simulink model "RL_multi_control_system"  (R2021a)
settings: Solver=ode23t  StartTime=0.0  StopTime=10.0  RelTol=1e-3  AbsTol=1e-3
undefined symbols (not defined in the file or in its folder): dphi0, dtheta0, phi0, Tf, theta0, Ts
libraries: angle_lib x8, rllib x2, simulink x2, pendulumLib x1
settings Model: DataDictionary=rl_data.sldd  Creator=tshintai  LastModifiedBy=THMOS
settings SolverCC: AutoScaleAbsTol=off
settings ExplorerConfigSet: InternalSimMechanicsExplorerSettings="<ExplorerConfiguration><canonicalview>default</canonicalview><AnimationSetting><BasePlaybackSpeed>1.0</BasePlaybackSpeed><PlaybackSpeedFactor>1.0</PlaybackSpeedFactor></AnimationSetting><TilePanel><TileInfo><Tiles Columns=\"1\" Count=\"1\" Rows=\"1\"><Column Weight=\"1\"/><Row Weight=\"1\"/><Tile Height=\"1\" Width=\"1\" X=\"0\" Y=\"0\"/></Tiles></TileInfo><SceneInfo><SceneViewer><BGColor><R>0.60000002384185791</R><G>0.60000002384185791</G><B>0.60000002384185791</B></BGColor><Camera><DoPerspective>on</DoPerspective><Position><X>0.334156231583514596</X><Y>0.107146061295956732</Y><Z>0.154419804164132285</Z></Position><Center><X>0.145480827141795971</X><Y>0.0537418892551446009</Y><Z>0.077934111254939889</Z></Center><Up><X>-0.332530024195597795</X><Y>-0.157027945704575345</Y><Z>0.929927958110882913</Z></Up><ViewLimDist>1</ViewLimDist><YLim>0.466307658154998583</YLim><XLim>0.535390274177961367</XLim></Camera></SceneViewer></SceneInfo></TilePanel><MechEditorPanel><Cameras><Camera><Id>Camera1</Id><Value><Name>Camera1</Name><NativeCamera><PositionKeyframeSet/><CenterKeyframeSet/><UpVectorKeyframeSet/></NativeCamera></Value></Camera></Cameras><GfxPanelCameraMap><MapElement CameraMLId=\"Camera1\" GfxPanelIndex=\"0\"/></GfxPanelCameraMap><VideoCreator><PlaybackSpeedRatio>1.0</PlaybackSpeedRatio><FrameRate>30</FrameRate><VideoFormat>Motion JPEG AVI</VideoFormat><FrameSize>auto</FrameSize></VideoCreator></MechEditorPanel></ExplorerConfiguration>"

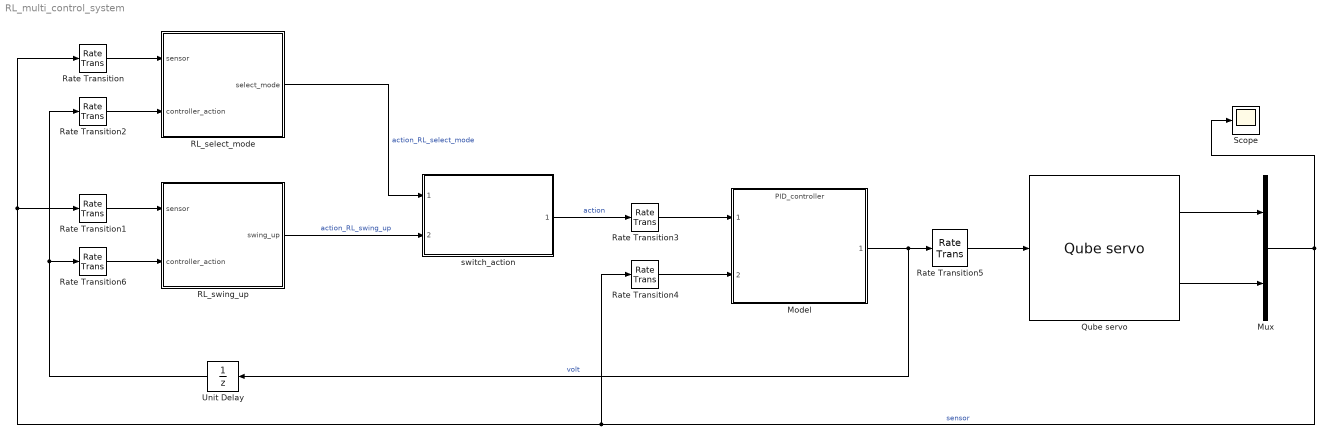
== system RL_multi_control_system ==
  Model : ModelReference  ModelNameDialog=PID_controller.slx  SimulationMode=Normal  ModelReferenceVersion=2.2
  Mux : Mux  Inputs=2
  Qube servo : pendulumLib/Qube servo  a0=[theta0, phi0]  w0=[dtheta0, dphi0]  R_m=R_m  L_m=L_m  mu_m=mu_m  K_b=K_b_2  n=n  rod_mass=m_r  rod_length=L_r  rod_rad=rod_rad  p_mass=m_p  p_length=L_p  p_rad=p_rad  D_r=D_r_2  D_p=D_p
  RL_select_mode : Subsystem
  RL_swing_up : Subsystem
  Rate Transition{,1..2,6} (4 alike) : RateTransition  OutPortSampleTime=Ts
  Rate Transition3 : RateTransition  OutPortSampleTime=Tc
  Rate Transition4 : RateTransition  OutPortSampleTime=Tc
  Rate Transition5 : RateTransition
  Scope : Scope
  Unit Delay : UnitDelay  SampleTime=-1  HasFrameUpgradeWarning=on
  switch_action : Subsystem  ReferencedSubsystem=RL_multi_switch_action
  wires:
  Qube servo/1 -> Mux/1
  Qube servo/2 -> Mux/2
  Mux/1 -> Rate Transition1/1, Rate Transition/1, Rate Transition4/1, Scope/1  "sensor"
  Rate Transition4/1 -> Model/2
  Model/1 -> Rate Transition5/1, Unit Delay/1  "volt"
  Rate Transition5/1 -> Qube servo/1
  Rate Transition3/1 -> Model/1
  Unit Delay/1 -> Rate Transition6/1, Rate Transition2/1
  RL_swing_up/1(swing_up) -> switch_action/2  "action_RL_swing_up"
  switch_action/1 -> Rate Transition3/1  "action"
  RL_select_mode/1(select_mode) -> switch_action/1  "action_RL_select_mode"
  Rate Transition/1 -> RL_select_mode/1(sensor)
  Rate Transition2/1 -> RL_select_mode/2(controller_action)
  Rate Transition1/1 -> RL_swing_up/1(sensor)
  Rate Transition6/1 -> RL_swing_up/2(controller_action)

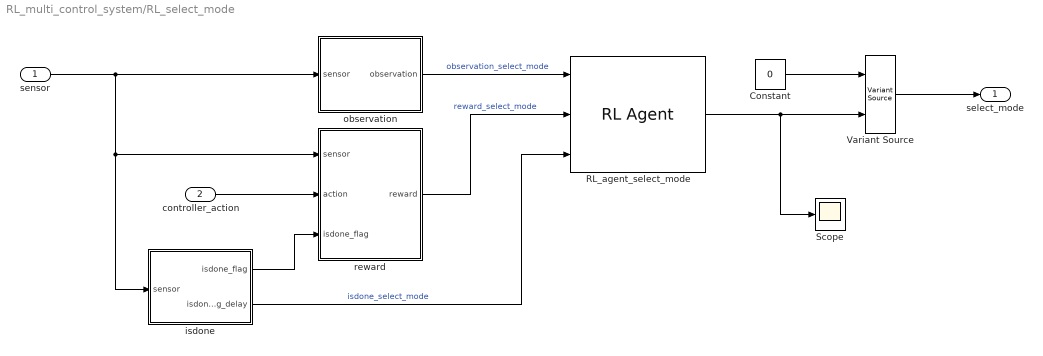
== system RL_multi_control_system/RL_select_mode ==
  sensor : Inport
  controller_action : Inport  Port=2
  Constant : Constant  Value=0
  RL_agent_select_mode : rllib/RL Agent  Agent=agent_select  ExternalActionAsInput=off  ProvideCumRwd=off  TreatAsDirectFeedthrough=on
  Scope : Scope
  Variant Source : VariantSource
  isdone : Subsystem  VariantControl=VARIANT_INV_POS
  "observation " : Subsystem  VariantControl=VARIANT_OBS_ARM_PEND
  reward : Subsystem  VariantControl=VARIANT_INV_POS
  select_mode : Outport
  wires:
  RL_agent_select_mode/1 -> Scope/1, Variant Source/2
  "observation "/1(observation) -> RL_agent_select_mode/1  "observation_select_mode"
  reward/1(reward) -> RL_agent_select_mode/2  "reward_select_mode"
  controller_action/1 -> reward/2(action)
  isdone/2(isdone_flag_delay) -> RL_agent_select_mode/3  "isdone_select_mode"
  sensor/1 -> "observation "/1(sensor), isdone/1(sensor), reward/1(sensor)
  isdone/1(isdone_flag) -> reward/3(isdone_flag)
  Variant Source/1 -> select_mode/1
  Constant/1 -> Variant Source/1

== system RL_multi_control_system/RL_swing_up ==
  sensor : Inport
  controller_action : Inport  Port=2
  Gain : Gain  Gain=3*pi/4
  RL_agent_swing_up : rllib/RL Agent  Agent=agent_swing  ExternalActionAsInput=off  ProvideCumRwd=off  TreatAsDirectFeedthrough=on
  isdone : Subsystem  VariantControl=VARIANT_INV_POS
  "observation " : Subsystem  VariantControl=VARIANT_OBS_ARM_PEND
  reward : Subsystem  VariantControl=VARIANT_INV_POS
  swing_up : Outport
  wires:
  isdone/1(isdone_flag) -> reward/3(isdone_flag)
  sensor/1 -> "observation "/1(sensor), isdone/1(sensor), reward/1(sensor)
  isdone/2(isdone_flag_delay) -> RL_agent_swing_up/3  "isdone_swing_up"
  controller_action/1 -> reward/2(action)
  reward/1(reward) -> RL_agent_swing_up/2  "reward_swing_up"
  "observation "/1(observation) -> RL_agent_swing_up/1  "observation_swing_up"
  RL_agent_swing_up/1 -> Gain/1
  Gain/1 -> swing_up/1

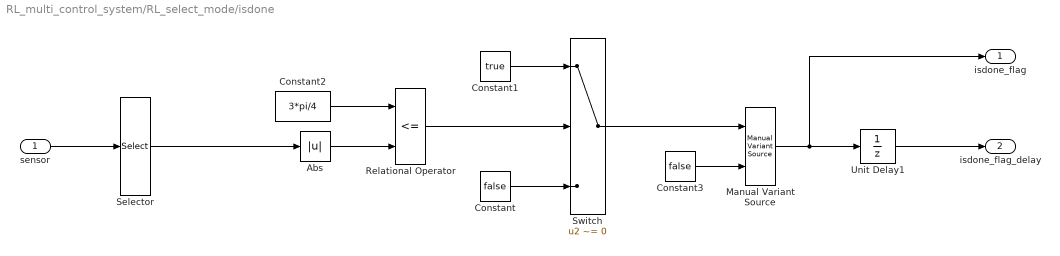
== system RL_multi_control_system/RL_select_mode/isdone ==
  sensor : Inport
  Abs : Abs
  Constant : Constant  Value=false
  Constant1 : Constant  Value=true
  Constant2 : Constant  Value=3*pi/4
  Constant3 : Constant  Value=false
  Manual Variant Source : simulink/Signal Routing/Manual Variant Source  NumChoices=2  LabelModeActiveChoice=V_2
  Relational Operator : RelationalOperator  Operator=<=  OutDataTypeStr=boolean  RndMeth=Simplest
  Selector : Selector  InputPortWidth=4  IndexOptions=Index vector (dialog)  Indices=[1]  OutputSizes=1
  Switch : Switch  Criteria=u2 ~= 0
  Unit Delay1 : UnitDelay  SampleTime=-1  HasFrameUpgradeWarning=on
  isdone_flag : Outport
  isdone_flag_delay : Outport  Port=2
  wires:
  Unit Delay1/1 -> isdone_flag_delay/1
  Constant3/1 -> Manual Variant Source/2
  Manual Variant Source/1 -> Unit Delay1/1, isdone_flag/1
  Switch/1 -> Manual Variant Source/1
  Selector/1 -> Abs/1
  Constant1/1 -> Switch/1
  Abs/1 -> Relational Operator/2
  Relational Operator/1 -> Switch/2
  Constant/1 -> Switch/3
  Constant2/1 -> Relational Operator/1
  sensor/1 -> Selector/1

== system RL_multi_control_system/RL_select_mode/observation  ==
  sensor : Inport
  Demux : Demux
  Mux : Mux  Inputs=6
  Trigonometric Function : Trigonometry
  Trigonometric Function1 : Trigonometry  Operator=cos
  Trigonometric Function2 : Trigonometry
  Trigonometric Function3 : Trigonometry  Operator=cos
  observation : Outport
  wires:
  Demux/3 -> Mux/5
  Demux/1 -> Trigonometric Function1/1, Trigonometric Function/1
  Trigonometric Function1/1 -> Mux/2
  Trigonometric Function/1 -> Mux/1
  Mux/1 -> observation/1  "observation"
  sensor/1 -> Demux/1
  Trigonometric Function2/1 -> Mux/3
  Trigonometric Function3/1 -> Mux/4
  Demux/2 -> Trigonometric Function3/1, Trigonometric Function2/1
  Demux/4 -> Mux/6

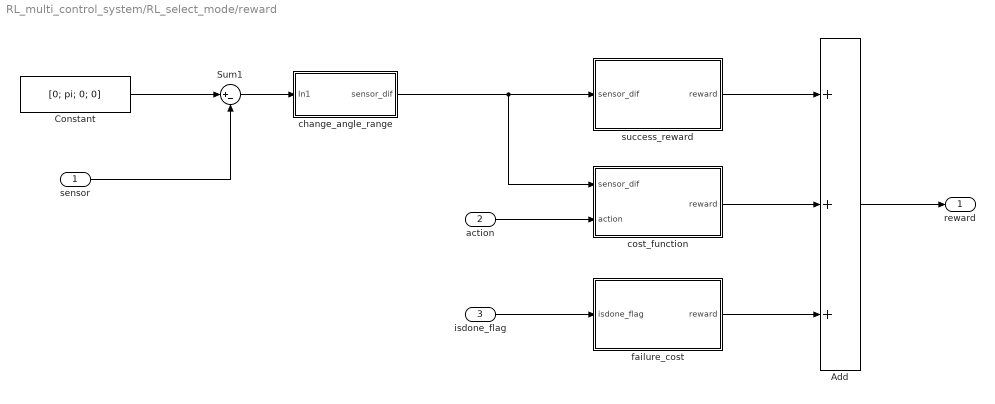
== system RL_multi_control_system/RL_select_mode/reward ==
  sensor : Inport
  action : Inport  Port=2
  isdone_flag : Inport  Port=3
  Add : Sum  Inputs=+++
  Constant : Constant  Value=[0; pi; 0; 0]
  Sum1 : Sum  Inputs=|+-
  change_angle_range : Subsystem
  cost_function : Subsystem
  failure_cost : Subsystem
  success_reward : Subsystem
  reward : Outport
  wires:
  isdone_flag/1 -> failure_cost/1(isdone_flag)
  failure_cost/1(reward) -> Add/3
  success_reward/1(reward) -> Add/1
  cost_function/1(reward) -> Add/2
  action/1 -> cost_function/2(action)
  Add/1 -> reward/1
  Sum1/1 -> change_angle_range/1(In1)
  sensor/1 -> Sum1/2
  Constant/1 -> Sum1/1
  change_angle_range/1(sensor_dif) -> success_reward/1(sensor_dif), cost_function/1(sensor_dif)

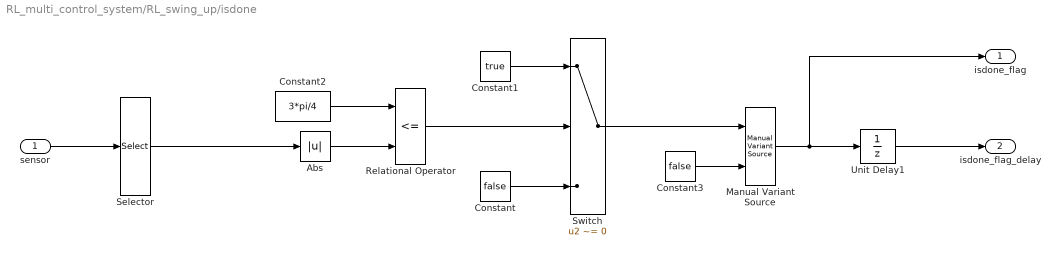
== system RL_multi_control_system/RL_swing_up/isdone ==
  sensor : Inport
  Abs : Abs
  Constant : Constant  Value=false
  Constant1 : Constant  Value=true
  Constant2 : Constant  Value=3*pi/4
  Constant3 : Constant  Value=false
  Manual Variant Source : simulink/Signal Routing/Manual Variant Source  NumChoices=2  LabelModeActiveChoice=V_2
  Relational Operator : RelationalOperator  Operator=<=  OutDataTypeStr=boolean  RndMeth=Simplest
  Selector : Selector  InputPortWidth=4  IndexOptions=Index vector (dialog)  Indices=[1]  OutputSizes=1
  Switch : Switch  Criteria=u2 ~= 0
  Unit Delay1 : UnitDelay  SampleTime=-1  HasFrameUpgradeWarning=on
  isdone_flag : Outport
  isdone_flag_delay : Outport  Port=2
  wires:
  sensor/1 -> Selector/1
  Constant2/1 -> Relational Operator/1
  Constant/1 -> Switch/3
  Relational Operator/1 -> Switch/2
  Abs/1 -> Relational Operator/2
  Constant1/1 -> Switch/1
  Selector/1 -> Abs/1
  Switch/1 -> Manual Variant Source/1
  Manual Variant Source/1 -> isdone_flag/1, Unit Delay1/1
  Constant3/1 -> Manual Variant Source/2
  Unit Delay1/1 -> isdone_flag_delay/1

== system RL_multi_control_system/RL_swing_up/observation  ==
  sensor : Inport
  Demux : Demux
  Mux : Mux  Inputs=6
  Trigonometric Function : Trigonometry
  Trigonometric Function1 : Trigonometry  Operator=cos
  Trigonometric Function2 : Trigonometry
  Trigonometric Function3 : Trigonometry  Operator=cos
  observation : Outport
  wires:
  Demux/4 -> Mux/6
  Demux/2 -> Trigonometric Function2/1, Trigonometric Function3/1
  Trigonometric Function3/1 -> Mux/4
  Trigonometric Function2/1 -> Mux/3
  sensor/1 -> Demux/1
  Mux/1 -> observation/1  "observation"
  Trigonometric Function/1 -> Mux/1
  Trigonometric Function1/1 -> Mux/2
  Demux/1 -> Trigonometric Function/1, Trigonometric Function1/1
  Demux/3 -> Mux/5

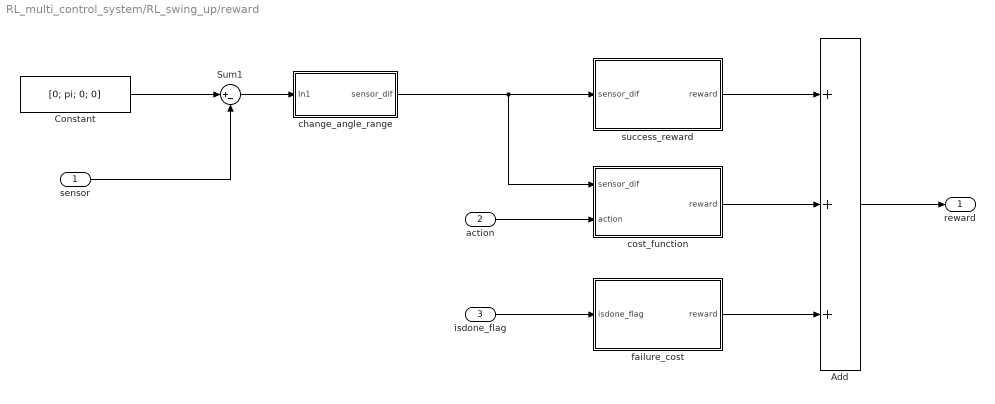
== system RL_multi_control_system/RL_swing_up/reward ==
  sensor : Inport
  action : Inport  Port=2
  isdone_flag : Inport  Port=3
  Add : Sum  Inputs=+++
  Constant : Constant  Value=[0; pi; 0; 0]
  Sum1 : Sum  Inputs=|+-
  change_angle_range : Subsystem
  cost_function : Subsystem
  failure_cost : Subsystem
  success_reward : Subsystem
  reward : Outport
  wires:
  isdone_flag/1 -> failure_cost/1(isdone_flag)
  failure_cost/1(reward) -> Add/3
  success_reward/1(reward) -> Add/1
  cost_function/1(reward) -> Add/2
  action/1 -> cost_function/2(action)
  Add/1 -> reward/1
  Sum1/1 -> change_angle_range/1(In1)
  sensor/1 -> Sum1/2
  Constant/1 -> Sum1/1
  change_angle_range/1(sensor_dif) -> success_reward/1(sensor_dif), cost_function/1(sensor_dif)

== system RL_multi_control_system/RL_select_mode/reward/change_angle_range ==
  In1 : Inport
  Demux : Demux
  Mux : Mux
  change_angle_range : angle_lib/change_angle_range  SystemSampleTime=-1  VariantActivationTime=update diagram  Latency=0  AutoFrameSizeCalculation=off
  change_angle_range1 : angle_lib/change_angle_range  SystemSampleTime=-1  VariantActivationTime=update diagram  Latency=0  AutoFrameSizeCalculation=off
  mod_2pi : angle_lib/mod_2pi  SystemSampleTime=-1  VariantActivationTime=update diagram  Latency=0  AutoFrameSizeCalculation=off
  mod_2pi1 : angle_lib/mod_2pi  SystemSampleTime=-1  VariantActivationTime=update diagram  Latency=0  AutoFrameSizeCalculation=off
  sensor_dif : Outport
  wires:
  mod_2pi1/1 -> change_angle_range1/1
  mod_2pi/1 -> change_angle_range/1
  Mux/1 -> sensor_dif/1
  Demux/4 -> Mux/4
  Demux/3 -> Mux/3
  change_angle_range1/1 -> Mux/2
  change_angle_range/1 -> Mux/1
  In1/1 -> Demux/1
  Demux/1 -> mod_2pi/1
  Demux/2 -> mod_2pi1/1

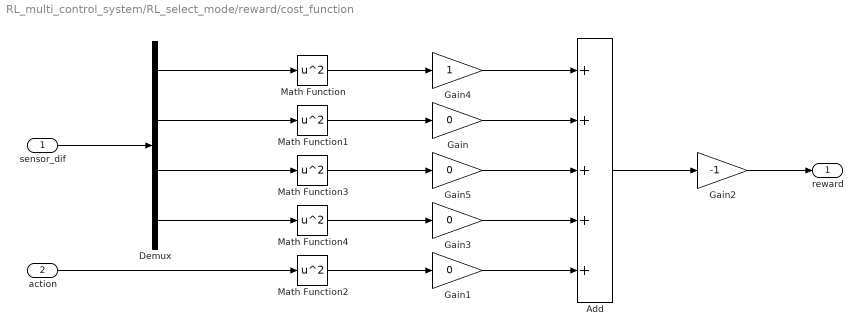
== system RL_multi_control_system/RL_select_mode/reward/cost_function ==
  sensor_dif : Inport
  action : Inport  Port=2
  Add : Sum  Inputs=+++++
  Demux : Demux
  Gain{,1,3,5} (4 alike) : Gain  Gain=0
  Gain2 : Gain  Gain=-1
  Gain4 : Gain
  Math Function{,1..4} (5 alike) : Math  Operator=square  SaturateOnIntegerOverflow=on
  reward : Outport
  wires:
  Math Function4/1 -> Gain3/1
  Gain4/1 -> Add/1
  Gain/1 -> Add/2
  Gain5/1 -> Add/3
  Gain3/1 -> Add/4
  Gain1/1 -> Add/5
  Gain2/1 -> reward/1
  Add/1 -> Gain2/1
  sensor_dif/1 -> Demux/1
  Demux/4 -> Math Function4/1
  Demux/3 -> Math Function3/1
  Demux/2 -> Math Function1/1
  Math Function1/1 -> Gain/1
  Math Function3/1 -> Gain5/1
  action/1 -> Math Function2/1
  Demux/1 -> Math Function/1
  Math Function/1 -> Gain4/1
  Math Function2/1 -> Gain1/1

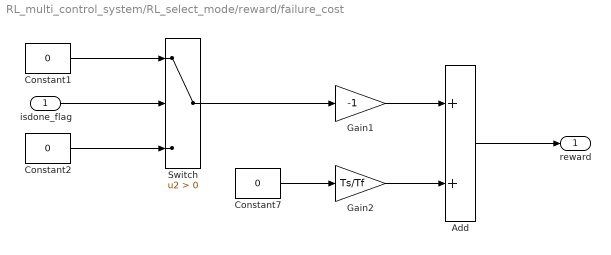
== system RL_multi_control_system/RL_select_mode/reward/failure_cost ==
  isdone_flag : Inport
  Add : Sum
  Constant1 : Constant  Value=0
  Constant2 : Constant  Value=0
  Constant7 : Constant  Value=0
  Gain1 : Gain  Gain=-1
  Gain2 : Gain  Gain=Ts/Tf
  Switch : Switch  Criteria=u2 > Threshold
  reward : Outport
  wires:
  Gain1/1 -> Add/1
  Constant2/1 -> Switch/3
  Constant1/1 -> Switch/1
  isdone_flag/1 -> Switch/2
  Switch/1 -> Gain1/1
  Gain2/1 -> Add/2
  Add/1 -> reward/1
  Constant7/1 -> Gain2/1

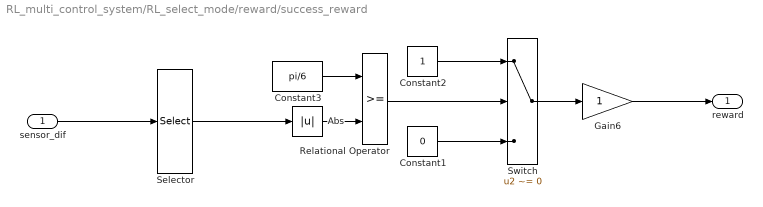
== system RL_multi_control_system/RL_select_mode/reward/success_reward ==
  sensor_dif : Inport
  Abs : Abs
  Constant1 : Constant  Value=0
  Constant2 : Constant
  Constant3 : Constant  Value=pi/6
  Gain6 : Gain
  Relational Operator : RelationalOperator  OutDataTypeStr=boolean  RndMeth=Simplest
  Selector : Selector  InputPortWidth=4  IndexOptions=Index vector (dialog)  Indices=[2]  OutputSizes=1
  Switch : Switch  Criteria=u2 ~= 0
  reward : Outport
  wires:
  sensor_dif/1 -> Selector/1
  Gain6/1 -> reward/1
  Selector/1 -> Abs/1
  Constant2/1 -> Switch/1
  Constant1/1 -> Switch/3
  Switch/1 -> Gain6/1
  Constant3/1 -> Relational Operator/1
  Abs/1 -> Relational Operator/2
  Relational Operator/1 -> Switch/2

== system RL_multi_control_system/RL_swing_up/reward/change_angle_range ==
  In1 : Inport
  Demux : Demux
  Mux : Mux
  change_angle_range : angle_lib/change_angle_range  SystemSampleTime=-1  VariantActivationTime=update diagram  Latency=0  AutoFrameSizeCalculation=off
  change_angle_range1 : angle_lib/change_angle_range  SystemSampleTime=-1  VariantActivationTime=update diagram  Latency=0  AutoFrameSizeCalculation=off
  mod_2pi : angle_lib/mod_2pi  SystemSampleTime=-1  VariantActivationTime=update diagram  Latency=0  AutoFrameSizeCalculation=off
  mod_2pi1 : angle_lib/mod_2pi  SystemSampleTime=-1  VariantActivationTime=update diagram  Latency=0  AutoFrameSizeCalculation=off
  sensor_dif : Outport
  wires:
  mod_2pi1/1 -> change_angle_range1/1
  mod_2pi/1 -> change_angle_range/1
  Mux/1 -> sensor_dif/1
  Demux/4 -> Mux/4
  Demux/3 -> Mux/3
  change_angle_range1/1 -> Mux/2
  change_angle_range/1 -> Mux/1
  In1/1 -> Demux/1
  Demux/1 -> mod_2pi/1
  Demux/2 -> mod_2pi1/1

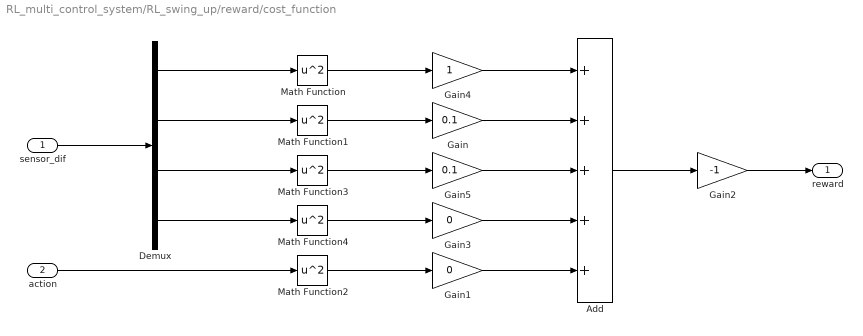
== system RL_multi_control_system/RL_swing_up/reward/cost_function ==
  sensor_dif : Inport
  action : Inport  Port=2
  Add : Sum  Inputs=+++++
  Demux : Demux
  Gain : Gain  Gain=0.1
  Gain1 : Gain  Gain=0
  Gain2 : Gain  Gain=-1
  Gain3 : Gain  Gain=0
  Gain4 : Gain
  Gain5 : Gain  Gain=0.1
  Math Function{,1..4} (5 alike) : Math  Operator=square  SaturateOnIntegerOverflow=on
  reward : Outport
  wires:
  Math Function4/1 -> Gain3/1
  Gain4/1 -> Add/1
  Gain/1 -> Add/2
  Gain5/1 -> Add/3
  Gain3/1 -> Add/4
  Gain1/1 -> Add/5
  Gain2/1 -> reward/1
  Add/1 -> Gain2/1
  sensor_dif/1 -> Demux/1
  Demux/4 -> Math Function4/1
  Demux/3 -> Math Function3/1
  Demux/2 -> Math Function1/1
  Math Function1/1 -> Gain/1
  Math Function3/1 -> Gain5/1
  action/1 -> Math Function2/1
  Demux/1 -> Math Function/1
  Math Function/1 -> Gain4/1
  Math Function2/1 -> Gain1/1

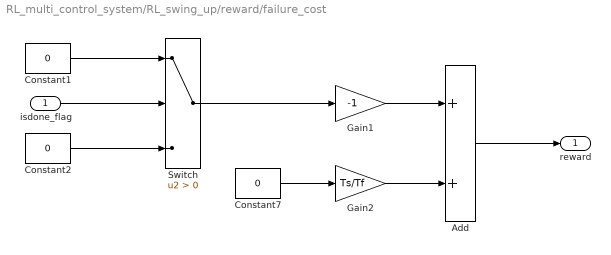
== system RL_multi_control_system/RL_swing_up/reward/failure_cost ==
  isdone_flag : Inport
  Add : Sum
  Constant1 : Constant  Value=0
  Constant2 : Constant  Value=0
  Constant7 : Constant  Value=0
  Gain1 : Gain  Gain=-1
  Gain2 : Gain  Gain=Ts/Tf
  Switch : Switch  Criteria=u2 > Threshold
  reward : Outport
  wires:
  Gain1/1 -> Add/1
  Constant2/1 -> Switch/3
  Constant1/1 -> Switch/1
  isdone_flag/1 -> Switch/2
  Switch/1 -> Gain1/1
  Gain2/1 -> Add/2
  Add/1 -> reward/1
  Constant7/1 -> Gain2/1

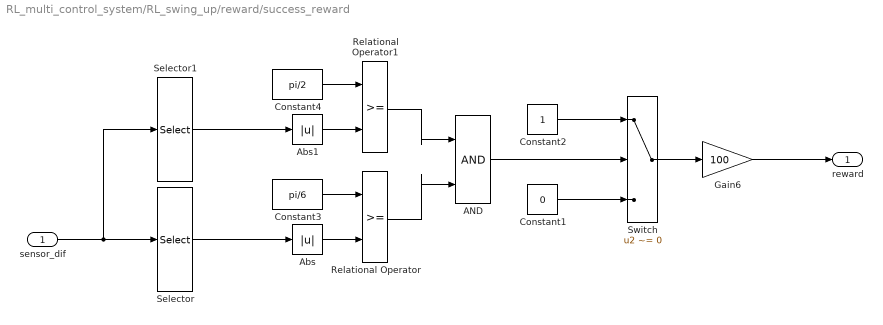
== system RL_multi_control_system/RL_swing_up/reward/success_reward ==
  sensor_dif : Inport
  AND : Logic  IconShape=distinctive  AllPortsSameDT=off  OutDataTypeStr=boolean
  Abs : Abs
  Abs1 : Abs
  Constant1 : Constant  Value=0
  Constant2 : Constant
  Constant3 : Constant  Value=pi/6
  Constant4 : Constant  Value=pi/2
  Gain6 : Gain  Gain=100
  Relational Operator : RelationalOperator  OutDataTypeStr=boolean  RndMeth=Simplest
  Relational Operator1 : RelationalOperator  OutDataTypeStr=boolean  RndMeth=Simplest
  Selector : Selector  InputPortWidth=4  IndexOptions=Index vector (dialog)  Indices=[2]  OutputSizes=1
  Selector1 : Selector  InputPortWidth=4  IndexOptions=Index vector (dialog)  Indices=[1]  OutputSizes=1
  Switch : Switch  Criteria=u2 ~= 0
  reward : Outport
  wires:
  sensor_dif/1 -> Selector1/1, Selector/1
  Gain6/1 -> reward/1
  Selector/1 -> Abs/1
  Constant2/1 -> Switch/1
  Constant1/1 -> Switch/3
  Switch/1 -> Gain6/1
  Constant3/1 -> Relational Operator/1
  Abs/1 -> Relational Operator/2
  AND/1 -> Switch/2
  Relational Operator/1 -> AND/2
  Abs1/1 -> Relational Operator1/2
  Constant4/1 -> Relational Operator1/1
  Relational Operator1/1 -> AND/1
  Selector1/1 -> Abs1/1
